simulink model "model"  (R2020b)
settings: Solver=VariableStepAuto  StartTime=0.0  StopTime=10.0  MaxStep=.001  RelTol=1e-3
model workspace (MAT data in the model file):
  Eb = Simulink.Parameter
  Eb.Value = 5
  Eb.DataType = 'auto'
  Eb.Dimensions = [1 1]
  L = Simulink.Parameter
  L.Value = 100
  L.DataType = 'auto'
  L.Dimensions = [1 1]
  Ra = Simulink.Parameter
  Ra.Value = 12
  Ra.DataType = 'auto'
  Ra.Dimensions = [1 1]
  Va = Simulink.Parameter
  Va.Value = 10
  Va.DataType = 'auto'
  Va.Dimensions = [1 1]
undefined symbols (not defined in the file): j, ke, kf, l, r
libraries: pid_lib x1
settings Model: OrderedModelArguments=off  Creator=SAGAR  LastModifiedBy=SAGAR

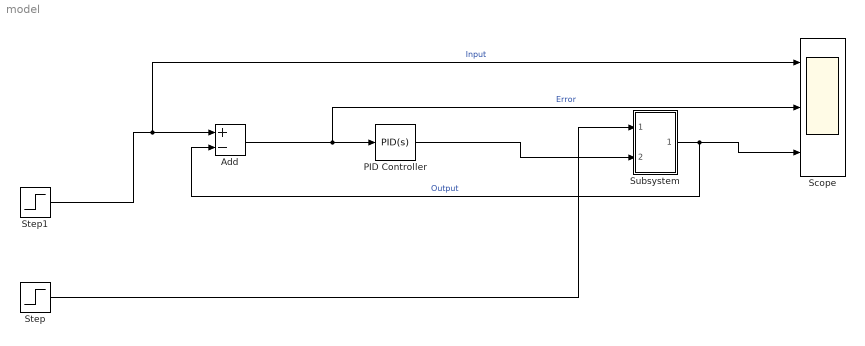
== system model ==
  Add : Sum  Inputs=+-
  PID Controller : pid_lib/PID Controller  Controller=PID  Form=Parallel  TimeDomain=Continuous-time  UseExternalTs=off  SampleTime=-1  IntegratorMethod=Forward Euler  FilterMethod=Forward Euler  ControllerParametersSource=internal  P=2.33732523131166  I=101.688590961822  D=-0.00216561164184195  UseFilter=on  N=391.307740793986  TunerSelectOption=Transfer Function Based (PID Tuner App)  InitialConditionSource=internal  InitialConditionForIntegrator=0  InitialConditionForFilter=0  DifferentiatorICPrevScaledInput=0  ExternalReset=none  TrackingMode=off  Kt=1  LimitOutput=off  SatLimitsSource=internal  UpperSaturationLimit=inf  LowerSaturationLimit=-inf  LinearizeAsGain=on  AntiWindupMode=none  Kb=1  POutMin=[]  POutMax=[]  IOutMin=[]  IOutMax=[]  DOutMin=[]  DOutMax=[]  NOutMin=[]  NOutMax=[]  SumOutMin=[]  SumOutMax=[]  SaturationOutMin=[]  SaturationOutMax=[]  PParamMin=[]  PParamMax=[]  IParamMin=[]  IParamMax=[]  DParamMin=[]  DParamMax=[]  NParamMin=[]  NParamMax=[]  KbParamMin=[]  KbParamMax=[]  KtParamMin=[]  KtParamMax=[]  KbOutMin=[]  KbOutMax=[]  KtOutMin=[]  KtOutMax=[]  IntegratorOutMin=[]  IntegratorOutMax=[]  FilterOutMin=[]  FilterOutMax=[]  SumI1OutMin=[]  SumI1OutMax=[]  SumI2OutMin=[]  SumI2OutMax=[]  SumI3OutMin=[]  SumI3OutMax=[]  SumI4OutMin=[]  SumI4OutMax=[]  SumDOutMin=[]  SumDOutMax=[]  DifferentiatorOutMin=[]  DifferentiatorOutMax=[]  FilterDiffOutCoefMin=[]  FilterDiffOutCoefMax=[]  ReciprocalOutMin=[]  ReciprocalOutMax=[]  SumDenOutMin=[]  SumDenOutMax=[]  SumNumOutMin=[]  SumNumOutMax=[]  DivideOutMin=[]  DivideOutMax=[]  UdiffTsProdOutMin=[]  UdiffTsProdOutMax=[]  NTsProdOutMin=[]  NTsProdOutMax=[]  UintegralTsProdOutMin=[]  UintegralTsProdOutMax=[]  UngainTsProdOutMin=[]  UngainTsProdOutMax=[]  IntegratorContinuousStateAttributes=''  IntegratorStateMustResolveToSignalObject=off  IntegratorRTWStateStorageClass=Auto  FilterContinuousStateAttributes=''  FilterStateMustResolveToSignalObject=off  FilterRTWStateStorageClass=Auto  ParallelPVariant=InternalParameters  IdealPVariant=Disabled  IVariant=InternalParameters  DVariant=InternalParameters  IntegratorVariant=Continuous  SatVariant=Disabled  AWVariant=Passthrough  PCopyVariant=Disabled  TRVariant=Disabled  FdbkBlocksVariant=Forward  IdealPFdbkVariant=Disabled  SatFdbkVariant=Disabled  DerivativeFilterVariant=ContFilter  NVariant=InternalParameters  NCopyVariant=Disabled  FilterICVariant=InternalICsFilter  IntegratorICVariant=InternalICs  ExternalResetVariant=Disabled  TRSumVariant=Passthrough  SumFdbkVariant=Disabled  SumVariant=Sum_PID  TsampFilterVariant=InternalTs  TsampNgainVariant=Passthrough  TsampIntegralVariant=Passthrough  ExternalSaturationOutDataTypeStr=Inherit: Same as second input
  Scope : Scope  NumInputPorts=3
  Step : Step  Time=2  After=-0.01  SampleTime=0
  Step1 : Step  SampleTime=0
  Subsystem : Subsystem
  wires:
  Add/1 -> Scope/2, PID Controller/1  "Error"
  PID Controller/1 -> Subsystem/2(In2)
  Step/1 -> Subsystem/1(In1)
  Step1/1 -> Scope/1, Add/1  "Input"
  Subsystem/1(Out1) -> Add/2, Scope/3  "Output"

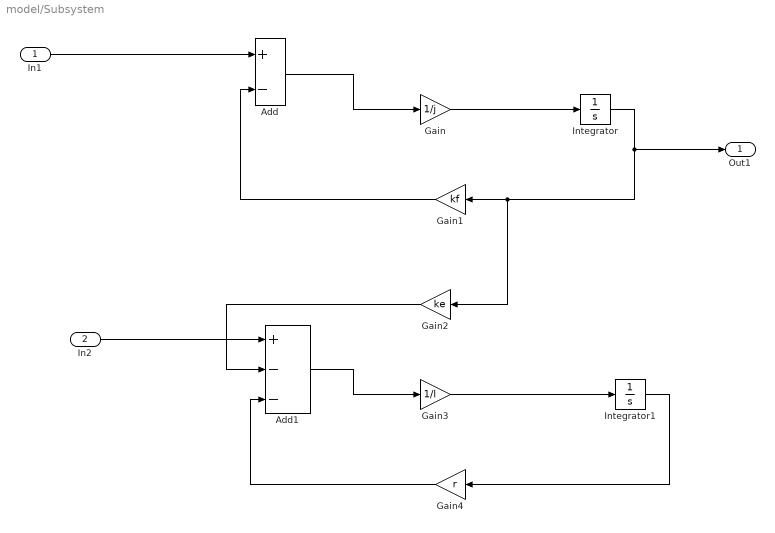
== system model/Subsystem ==
  In1 : Inport
  In2 : Inport  Port=2
  Add : Sum  Inputs=+-
  Add1 : Sum  Inputs=+--
  Gain : Gain  Gain=1/j
  Gain1 : Gain  Gain=kf
  Gain2 : Gain  Gain=ke
  Gain3 : Gain  Gain=1/l
  Gain4 : Gain  Gain=r
  Integrator : Integrator
  Integrator1 : Integrator
  Out1 : Outport
  wires:
  Integrator/1 -> Out1/1, Gain2/1, Gain1/1
  Gain3/1 -> Integrator1/1
  Gain4/1 -> Add1/3
  Gain2/1 -> Add1/2
  Gain1/1 -> Add/2
  Gain/1 -> Integrator/1
  Add1/1 -> Gain3/1
  Integrator1/1 -> Gain4/1
  Add/1 -> Gain/1
  In2/1 -> Add1/1
  In1/1 -> Add/1
